simulink model "CSvRTHS_Client"  (R2020b)
settings: Solver=ode8  StartTime=0.0  StopTime=inf  FixedStep=samplePeriod  RelTol=1e-3  AbsTol=1e-6  EnableMultiTasking=on
PreLoadFcn:
  | initializeSimulation;
InitFcn:
  | clear('all');
  | initializeSimulation;
values from neighbouring files (symbols this model uses):
  adaptivegain = diag(10.^[6.03 4.23 1.48 -1.10])    [initializeSimulation.m]
  Area = 0.751    [initializeSimulation.m]
  Be = 95958    [initializeSimulation.m]
  Cl = 5.89e-6    (= 5.89e-06)    [initializeSimulation.m]
  coef = 1.0    (= 1)    [initializeSimulation.m]
  damperB = 0    [initializeSimulation.m]
  damperCanon = 1    [initializeSimulation.m]
  Derivadas = [u;dudt;dudt2;dudt3]    [initializeSimulation.m]
  forceCanon = 1    [initializeSimulation.m]
  frictionB = 0    [initializeSimulation.m]
  Gsnsr_DT = 1    [initializeSimulation.m]
  Gsnsr_FT = 1    [initializeSimulation.m]
  Kc = 1.36e-5    (= 1.36e-05)    [initializeSimulation.m]
  Kp = 3.0    (= 3)    [initializeSimulation.m]
  Kq = 23.01    [initializeSimulation.m]
  kv = 1    [initializeSimulation.m]
  lengthCanon = 1    [initializeSimulation.m]
  max_amb = [amb0max,amb1max,amb2max,amb3max]*1e15    [initializeSimulation.m]
  maxDisplB = (stroke2B + endLength2B) * lengthCanon    (= 42)    [initializeSimulation.m]
  maxVelocB = (maxFlowB * flowCanon / (area1B * areaCanon)) / velocCanon    [initializeSimulation.m]
  me = 0.023/1000    (= 2.3e-05)    [initializeSimulation.m]
  min_amb = [amb0min,amb1min,amb2min,amb3min]    [initializeSimulation.m]
  minDisplB = -(stroke1B + endLength1B) * lengthCanon    (= -42)    [initializeSimulation.m]
  minVelocB = -(maxFlowB * flowCanon / (area2B * areaCanon)) / velocCanon    [initializeSimulation.m]
  samplePeriod = 0.5/1024    (= 0.00048828125)    [initializeSimulation.m]
  sat_limit_lower = -3.8    [initializeSimulation.m]
  sat_limit_upper = +3.8    (= 3.8)    [initializeSimulation.m]
  Seed_snr = rng(seed)    [initializeSimulation.m]
  staticForceB = 0    [initializeSimulation.m]
  tauv = 0.00332    [initializeSimulation.m]
  velocCanon = 1    [initializeSimulation.m]
  Vt = 48.66    [initializeSimulation.m]
  yieldDisplB = 0.1    [initializeSimulation.m]
undefined symbols (not defined in the file or in its folder): denfilter, DiscIntNeverNeededParam, HybridCtrlParameters, numfilter
libraries: simulink x7, dsparch4 x1, sldrtlib x1
settings Model: ExtModeTrigMode=oneshot  ExtModeArmWhenConnect=off  ExtModeAutoUpdateStatusClock=off  Creator=Andreas Schellenberg  LastModifiedBy=diego.mera
settings SolverCC: AutoScaleAbsTol=off
settings DataIOCC: LimitDataPoints=on  SaveFormat=Array  SaveOutput=off  ReturnWorkspaceOutputs=off  SignalLoggingName=sigsOut
settings OptimizationCC: ExpressionDepthLimit=2147483647  InitFltsAndDblsToZero=on  LifeSpan=inf
settings DebuggingCC: SaveWithParameterizedLinksMsg=none  CheckSSInitialOutputMsg=off  UnderspecifiedInitializationDetection=Classic  MergeDetectMultiDrivingBlocksExec=none  MultiTaskDSMMsg=warning  MultiTaskCondExecSysMsg=none  StateNameClashWarn=warning  SFUnexpectedBacktrackingDiag=warning  SFNoUnconditionalDefaultTransitionDiag=warning  SFExecutionAtInitializationDiag=none  ArithmeticOperatorsInVariantConditions=warning
settings HardwareCC: ProdBitPerPointer=32  ProdBitPerSizeT=32  ProdBitPerPtrDiffT=32  ProdLargestAtomicFloat=None  ProdIntDivRoundTo=Undefined  ProdEndianess=Unspecified  ProdWordSize=32  ProdHWDeviceType=32-bit Generic  TargetUnknown=on
settings ModelReferenceCC: PropagateSignalLabelsOutOfModel=off
settings SFSimCC: SimCustomHeaderCode="#include \"PredictorCorrector.h\""  SimUserSources=PredictorCorrector.c  SimUseLocalCustomCode=off  SimParseCustomCode=off  CustomCodeUndefinedFunction=UseInterfaceOnly
settings RTWCC: RTWUseLocalCustomCode=off
settings CodeAppCC: StateflowObjectComments=on
settings GRTTargetCC: TargetFcnLib=ansi_tfl_tmw.mat  TargetLangStandard=C89/C90 (ANSI)  CombineOutputUpdateFcns=off  GRTInterface=on
settings ConfigComp: CovMetricSettings=dw  CovSaveCumulativeToWorkspaceVar=on  CovSaveSingleToWorkspaceVar=on  CovExternalEMLEnable=off  CovSFcnEnable=off

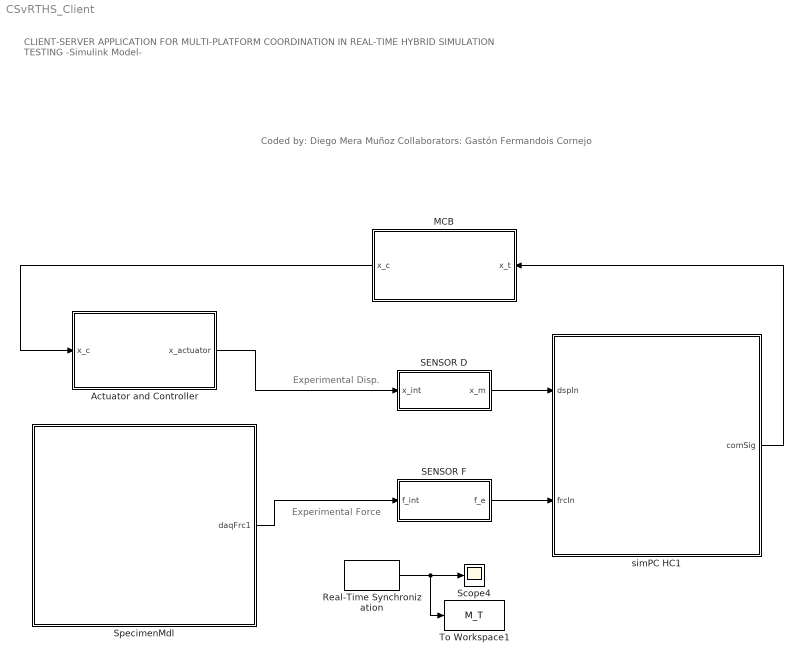
== system CSvRTHS_Client ==
  note: CLIENT-SERVER APPLICATION FOR MULTI-PLATFORM COORDINATION IN REAL-TIME HYBRID SIMULATION TESTING
      | -Simulink Model-
  note: Coded by: Diego Mera Muñoz
      | Collaborators: Gastón Fermandois Cornejo
  note: Experimental Force
  note: Experimental Disp.
  Actuator and Controller : Subsystem
      mask Display: disp('ACTUATOR\nMODEL')
  MCB : Subsystem
      mask Display: disp('ADAPTIVE\nMODEL-BASED\nCOMPENSATION')
  Real-Time Synchronization : sldrtlib/Real-Time Synchronization  SampleTime=0.5/1024  MaxMissedTicks=1000000  ShowMissedTicks=on  YieldWhenWaiting=off
  SENSOR D : Subsystem
  SENSOR F : Subsystem
  Scope4 : Scope
  SpecimenMdl : Subsystem
      mask Display: disp('EXPERIMENTAL\nSUBSTRUCTURE')
  To Workspace1 : ToWorkspace  VariableName=M_T  SaveFormat=Timeseries  SampleTime=-1
  simPC HC1 : Subsystem  mask(Hybrid Controller: D2/D2){nDOF=HybridCtrlParameters.nDOF, upFact=HybridCtrlParameters.upFact, dtInt=HybridCtrlParameters.dtInt, dtSim=HybridCtrlParameters.dtSim, dtCon=HybridCtrlParameters.dtCon, N=HybridCtrlParameters.N, iDelay=HybridCtrlParameters.iDelay}
      mask prompts: nDOF "Number of DOF: nDOF"; upFact "Upsample Factor: upFact"; dtInt "Integration time step: dtInt"; dtSim "Simulation time step: dtSim"; dtCon "Controller time step: dtCon"; N "Number of substeps: N"; iDelay "Number of delay steps: iDelay"
      mask help: Hybrid Controller using C0-continuous quadratic Lagrange interpolation for prediction and correction
      mask Display: disp('NUMERICAL\nSUBSTRUCTURE')
  wires:
  SENSOR F/1("f_e ") -> simPC HC1/2(frcIn)
  MCB/1(x_c) -> Actuator and Controller/1(x_c)
  SpecimenMdl/1(daqFrc1) -> SENSOR F/1(f_int)
  SENSOR D/1(x_m) -> simPC HC1/1(dspIn)
  simPC HC1/1(comSig) -> MCB/1(x_t)
  Actuator and Controller/1(x_actuator) -> SENSOR D/1(x_int)
  Real-Time Synchronization/1 -> To Workspace1/1, Scope4/1

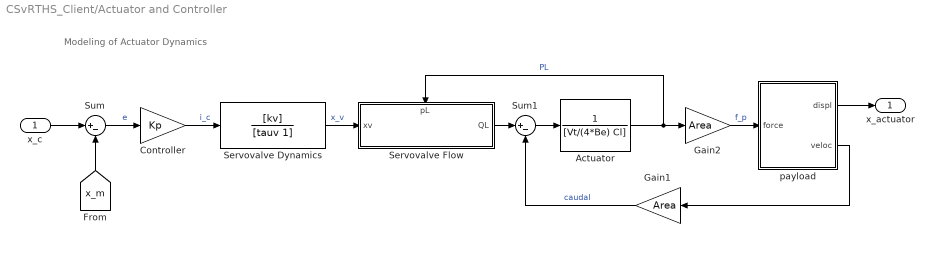
== system CSvRTHS_Client/Actuator and Controller ==
  note: Modeling of Actuator Dynamics
  x_c : Inport
  Actuator : TransferFcn  Denominator=[Vt/(4*Be) Cl]
      mask Display: image(imread('actuator.PNG'));
  Controller : Gain  Gain=Kp
  Gain1 : Gain  Gain=Area
  Gain2 : Gain  Gain=Area
  Servovalve Dynamics : TransferFcn  Numerator=[kv]  Denominator=[tauv 1]
      mask Display: image(imread('servo2.PNG'));
  Servovalve Flow : Subsystem
      settings: PortSchema="{\"entries\":[{\"content\":{\"sides\":[{\"content\":{\"connectorIds\":[\"In1\"]},\"type\":\"ConnectorPlacement.EquallySpacedRectSide\",\"uuid\":\"f3a8b7d5-d784-462c-bc82-60644eee5a75\"},{\"content\":{\"connectorIds\":[\"Out1\"],\"side\":\"RIGHT\"},\"type\":\"ConnectorPlacement.EquallySpacedRectSide\",\"uuid\":\"5e6f1f83-a632-4bc9-a761-43cae998e77f\"},{\"content\":{\"connectorIds\":[\"In2\"],\"side\":\"TOP\"},\"type\":\"ConnectorPlacement.EquallySpacedRectSide\",\"uuid\":\"989b0903-e260-4847-946f-0ac5d5e511f7\"}]},\"type\":\"ConnectorPlacement.EquallySpacedConnector\",\"uuid\":\"5619e211-faa3-4076-b1a0-b20862ba0eaa\"}],\"packageUris\":[\"http://schema.mathworks.com/mf0/Connector/19700101\"],\"version\":\"1.0\"}"
      mask Display: image(imread('servo.PNG'));
  Sum : Sum  Inputs=|+-
  Sum1 : Sum  Inputs=|+-
  payload : Subsystem
  x_actuator : Outport  VectorParamsAs1DForOutWhenUnconnected=off
  wires:
  Sum1/1 -> Actuator/1
  Sum/1 -> Controller/1  "e"
  Servovalve Dynamics/1 -> Servovalve Flow/1(xv)  "x_v"
  Servovalve Flow/1(QL) -> Sum1/1
  Gain1/1 -> Sum1/2  "caudal"
  Actuator/1 -> Gain2/1, Servovalve Flow/2(pL)  "PL"
  payload/1(displ) -> x_actuator/1
  Controller/1 -> Servovalve Dynamics/1  "i_c"
  payload/2(veloc) -> Gain1/1
  Gain2/1 -> payload/1(force)  "f_p"
  x_c/1 -> Sum/1
  [x_m] -> Sum/2

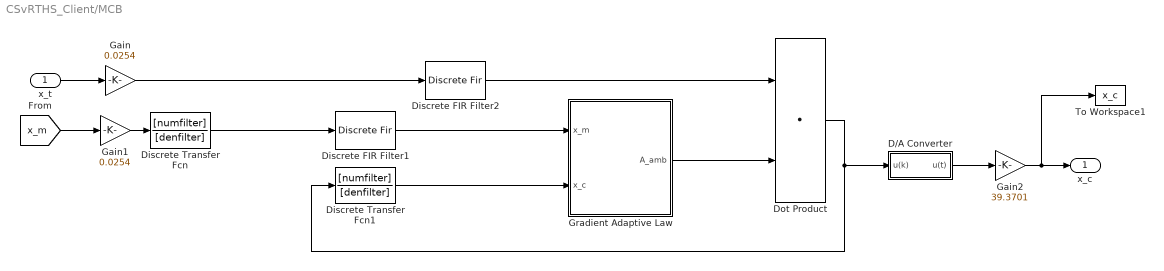
== system CSvRTHS_Client/MCB ==
  x_t : Inport
  D/A Converter : Subsystem
  Discrete Transfer Fcn : DiscreteTransferFcn  Numerator=[numfilter]  Denominator=[denfilter]
  Discrete Transfer Fcn1 : DiscreteTransferFcn  Numerator=[numfilter]  Denominator=[denfilter]
  Discrete FIR Filter1 : DiscreteFir  Coefficients=Derivadas
  Discrete FIR Filter2 : DiscreteFir  Coefficients=Derivadas
  Dot Product : DotProduct  InputSameDT=on  OutDataTypeStr=Inherit: Inherit via internal rule
  Gain : Gain  Gain=0.0254
  Gain1 : Gain  Gain=0.0254
  Gain2 : Gain  Gain=39.3701
  Gradient Adaptive Law : Subsystem
  To Workspace1 : ToWorkspace  VariableName=x_c  SaveFormat=Timeseries  SampleTime=-1
  x_c : Outport  VectorParamsAs1DForOutWhenUnconnected=off
  wires:
  Gradient Adaptive Law/1(A_amb) -> Dot Product/2
  Discrete FIR Filter1/1 -> Gradient Adaptive Law/1(x_m)
  Discrete Transfer Fcn1/1 -> Gradient Adaptive Law/2(x_c)
  [x_m] -> Gain1/1
  Discrete Transfer Fcn/1 -> Discrete FIR Filter1/1
  x_t/1 -> Gain/1
  Dot Product/1 -> D/A Converter/1(u(k)), Discrete Transfer Fcn1/1
  Discrete FIR Filter2/1 -> Dot Product/1
  D/A Converter/1(u(t)) -> Gain2/1
  Gain1/1 -> Discrete Transfer Fcn/1
  Gain/1 -> Discrete FIR Filter2/1
  Gain2/1 -> To Workspace1/1, x_c/1

== system CSvRTHS_Client/SENSOR D ==
  x_int : Inport
  Sensor Noise : simulink/Sources/Band-Limited White Noise  Cov=rms_noise_DT  Ts=samplePeriod  seed=double(Seed_snr.Seed)
  Sensor Gain LVDT : Gain  Gain=Gsnsr_DT  SaturateOnIntegerOverflow=on  OutDataTypeStr=Inherit: Same as input  ParamDataTypeStr=Inherit: Same as input
  Sum : Sum  Inputs=|++  InputSameDT=on  SaturateOnIntegerOverflow=on  OutDataTypeStr=Inherit: Same as first input
  To Workspace : ToWorkspace  VariableName=x_m  SaveFormat=Timeseries  SampleTime=-1
  x_m : Outport
  tag scope: x_m=global
  wires:
  Sensor Gain LVDT/1 -> Sum/1
  Sensor Noise/1 -> Sum/2
  x_int/1 -> Sensor Gain LVDT/1
  Sum/1 -> [x_m], x_m/1, To Workspace/1

== system CSvRTHS_Client/SENSOR F ==
  f_int : Inport
  Sensor Noise1 : simulink/Sources/Band-Limited White Noise  Cov=rms_noise_FT  Ts=samplePeriod  seed=double(Seed_snr.Seed)
  Sensor Gain LOAD CELL : Gain  Gain=Gsnsr_FT  SaturateOnIntegerOverflow=on  OutDataTypeStr=Inherit: Same as input  ParamDataTypeStr=Inherit: Same as input
  Sum1 : Sum  Inputs=|++  InputSameDT=on  SaturateOnIntegerOverflow=on  OutDataTypeStr=Inherit: Same as first input
  To Workspace1 : ToWorkspace  VariableName=f_m  SaveFormat=Timeseries  SampleTime=-1
  "f_e " : Outport
  wires:
  Sensor Gain LOAD CELL/1 -> Sum1/1
  Sum1/1 -> To Workspace1/1, "f_e "/1
  Sensor Noise1/1 -> Sum1/2
  f_int/1 -> Sensor Gain LOAD CELL/1

== system CSvRTHS_Client/SpecimenMdl ==
  note: Experimental Force
  note: Experimental Disp
  S-Function : S-Function  FunctionName=SFun_GenericClient  Parameters=ipAddr,ipPort,dataSize  SFunctionDeploymentMode=off  EnableBusSupport=off  mask(GenericClient Element){ipAddr=127.0.0.1, ipPort=8093, dataSize=256}
      mask prompts: ipAddr "IP Address of Server"; ipPort "IP Port Number of Server"; dataSize "Size of Data Arrays"
      mask Display: disp('GenericClient\nElement');
  Scope1 : Scope
  Terminator1 : Terminator
  daqFrc1 : Outport
  tag scope: ch3b=global
  wires:
  [ch3a] -> S-Function/1
  S-Function/1 -> Terminator1/1
  S-Function/2 -> daqFrc1/1, [ch3b], Scope1/1

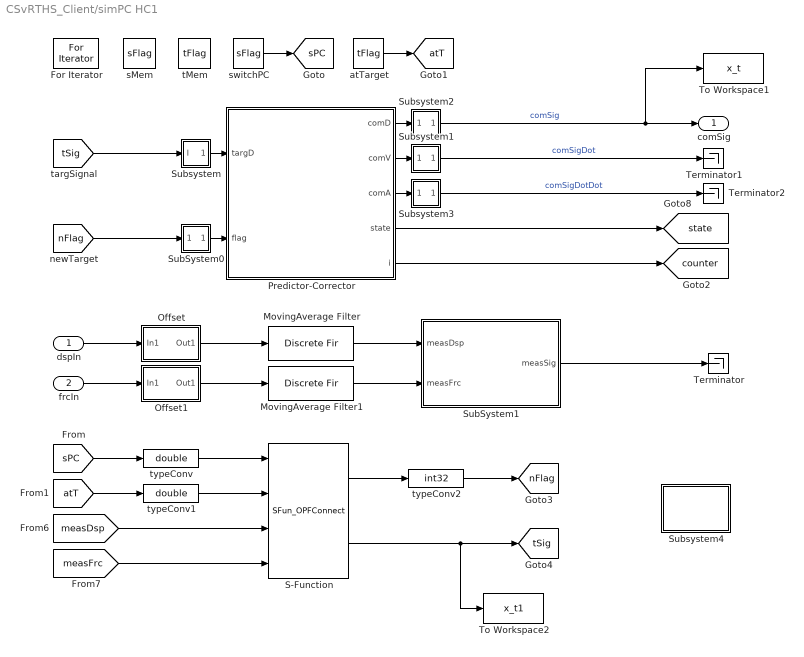
== system CSvRTHS_Client/simPC HC1 ==
  dspIn : Inport
  frcIn : Inport  Port=2
  For Iterator : ForIterator  IterationLimit=upFact  ShowIterationPort=off
  MovingAverage Filter : DiscreteFir  Coefficients=1/numSample*ones(1,numSample)  mask(Moving Average Filter){numSample=1}
      mask prompts: numSample "Number of Samples: numSample"
      mask help:
      | Moving average filter by using discrete FIR filter.
      | Set numSample = 1 for no filtering.
      mask Display: fprintf('MovingAverage\nFilter')
  MovingAverage Filter1 : DiscreteFir  Coefficients=1/numSample*ones(1,numSample)  mask(Moving Average Filter){numSample=1}
      mask prompts: numSample "Number of Samples: numSample"
      mask help:
      | Moving average filter by using discrete FIR filter.
      | Set numSample = 1 for no filtering.
      mask Display: fprintf('MovingAverage\nFilter')
  Offset : Subsystem  mask(Signal Offset){nS=nDOF, nOffset=-1}
      mask prompts: nS "Number of Signals: nS"; nOffset "Number of samples to initialize offset: nOffset"
      mask help:
      | Offset signal by average of signal over initial number of samples.
      | Set nOffset = -1 for no signal offset.
      mask Display: fprintf('Signal\nOffset')
  Offset1 : Subsystem  mask(Signal Offset){nS=nDOF, nOffset=-1}
      mask prompts: nS "Number of Signals: nS"; nOffset "Number of samples to initialize offset: nOffset"
      mask help:
      | Offset signal by average of signal over initial number of samples.
      | Set nOffset = -1 for no signal offset.
      mask Display: fprintf('Signal\nOffset')
  Predictor-Corrector : Stateflow chart  TreatAsAtomicUnit=on
  S-Function : S-Function  FunctionName=SFun_OPFConnect  Parameters=ipPort  SFunctionDeploymentMode=off  EnableBusSupport=off  mask(OpenFresco Connect){ipPort=8090}
      mask prompts: ipPort "IP Port Number of Server"
      mask Display: disp('OpenFresco\nConnect');
  SubSystem0 : Subsystem
      mask Display: disp('I/O')
  SubSystem1 : Subsystem
  Subsystem : Subsystem
      mask Display: disp('I/O')
  Subsystem1 : Subsystem
      mask Display: disp('I/O')
  Subsystem2 : Subsystem
      mask Display: disp('I/O')
  Subsystem3 : Subsystem
      mask Display: disp('I/O')
  Subsystem4 : Subsystem
      mask Display: disp('Scopes')
  Terminator : Terminator
  Terminator1 : Terminator
  Terminator2 : Terminator
  To Workspace1 : ToWorkspace  VariableName=x_t  SaveFormat=Timeseries  SampleTime=-1
  To Workspace2 : ToWorkspace  VariableName=x_t1  SaveFormat=Timeseries  SampleTime=-1
  atTarget : DataStoreRead  DataStoreName=tFlag
  sMem : DataStoreMemory  DataStoreName=sFlag  ShowAdditionalParam=off  OutDataTypeStr=int32
  switchPC : DataStoreRead  DataStoreName=sFlag
  tMem : DataStoreMemory  DataStoreName=tFlag  ShowAdditionalParam=off  OutDataTypeStr=int32
  typeConv : DataTypeConversion  OutDataTypeStr=double  RndMeth=Round  SaturateOnIntegerOverflow=on
  typeConv1 : DataTypeConversion  OutDataTypeStr=double  RndMeth=Round  SaturateOnIntegerOverflow=on
  typeConv2 : DataTypeConversion  OutDataTypeStr=int32  RndMeth=Round  SaturateOnIntegerOverflow=on
  comSig : Outport
  tag scope: atT=global, counter=global, nFlag=global, sPC=global, state=global, tSig=global
  wires:
  SubSystem0/1(Out) -> Predictor-Corrector/2(flag)
  [nFlag] -> SubSystem0/1(In)
  [tSig] -> Subsystem/1(I)
  [sPC] -> typeConv/1
  [atT] -> typeConv1/1
  S-Function/1 -> typeConv2/1
  S-Function/2 -> [tSig], To Workspace2/1
  Subsystem/1(O) -> Predictor-Corrector/1(targD)
  Subsystem2/1(Out) -> comSig/1, To Workspace1/1  "comSig"
  switchPC/1 -> [sPC]
  atTarget/1 -> [atT]
  Predictor-Corrector/1(comD) -> Subsystem2/1(In)
  Subsystem1/1(Out) -> Terminator1/1  "comSigDot"
  Predictor-Corrector/2(comV) -> Subsystem1/1(In)
  Subsystem3/1(Out) -> Terminator2/1  "comSigDotDot"
  Predictor-Corrector/3(comA) -> Subsystem3/1(In)
  frcIn/1 -> Offset1/1(In1)
  SubSystem1/1(measSig) -> Terminator/1
  dspIn/1 -> Offset/1(In1)
  MovingAverage Filter/1 -> SubSystem1/1(measDsp)
  MovingAverage Filter1/1 -> SubSystem1/2(measFrc)
  Offset/1(Out1) -> MovingAverage Filter/1
  Offset1/1(Out1) -> MovingAverage Filter1/1
  Predictor-Corrector/5(i) -> [counter]
  Predictor-Corrector/4(state) -> [state]
  [measFrc] -> S-Function/4
  [measDsp] -> S-Function/3
  typeConv/1 -> S-Function/1
  typeConv1/1 -> S-Function/2
  typeConv2/1 -> [nFlag]

== system CSvRTHS_Client/Actuator and Controller/Servovalve Flow ==
  xv : Inport
  pL : Inport  Port=2
  Gain : Gain  Gain=Kq
  Gain1 : Gain  Gain=Kc
  Subtract : Sum  Inputs=+-
  QL : Outport
  wires:
  Gain1/1 -> Subtract/2
  pL/1 -> Gain1/1
  Subtract/1 -> QL/1
  Gain/1 -> Subtract/1
  xv/1 -> Gain/1

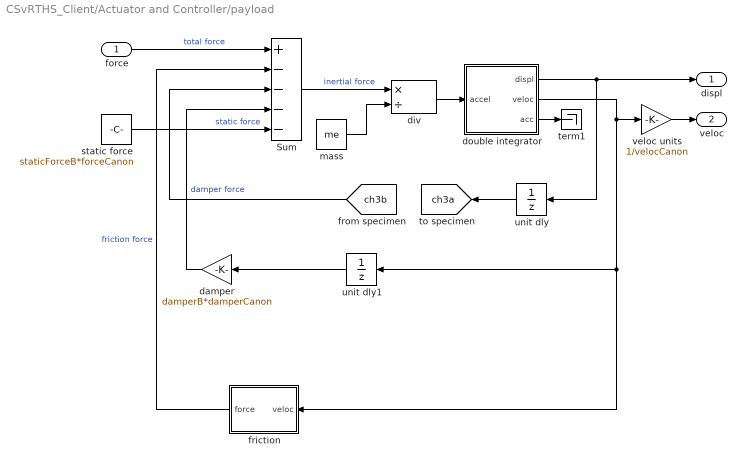
== system CSvRTHS_Client/Actuator and Controller/payload ==
  force : Inport
  Sum : Sum  Inputs=+----  InputSameDT=on  SaturateOnIntegerOverflow=on  OutDataTypeStr=Inherit: Same as first input
  damper : Gain  Gain=damperB*damperCanon  SaturateOnIntegerOverflow=on  OutDataTypeStr=Inherit: Same as input  ParamDataTypeStr=Inherit: Same as input
  div : Product  Inputs=*/  InputSameDT=on  SaturateOnIntegerOverflow=on  OutDataTypeStr=Inherit: Same as first input
  double integrator : Subsystem
  friction : Subsystem  mask{friction=frictionB*forceCanon, yieldDispl=yieldDisplB*lengthCanon, hysteresis=0}
      mask prompts: friction "Sliding friction"; yieldDispl "Equiv. yield displacement (in)"; hysteresis "Hysteresis constant"
  mass : Constant  Value=me
  static force : Constant  Value=staticForceB*forceCanon
  term1 : Terminator
  unit dly : UnitDelay  SampleTime=-1  HasFrameUpgradeWarning=on
  unit dly1 : UnitDelay  SampleTime=-1  HasFrameUpgradeWarning=on
  veloc units : Gain  Gain=1/velocCanon  SaturateOnIntegerOverflow=on  OutDataTypeStr=Inherit: Same as input  ParamDataTypeStr=Inherit: Same as input
  displ : Outport
  veloc : Outport  Port=2
  tag scope: ch3a=global
  wires:
  unit dly1/1 -> damper/1
  unit dly/1 -> [ch3a]
  damper/1 -> Sum/4  "damper force"
  static force/1 -> Sum/5  "static force"
  double integrator/2(veloc) -> unit dly1/1, friction/1(veloc), veloc units/1
  double integrator/1(displ) -> unit dly/1, displ/1
  div/1 -> double integrator/1(accel)
  double integrator/3(acc) -> term1/1
  mass/1 -> div/2
  force/1 -> Sum/1  "total force"
  Sum/1 -> div/1  "inertial force"
  veloc units/1 -> veloc/1
  friction/1(force) -> Sum/2  "friction force"
  [ch3b] -> Sum/3

== system CSvRTHS_Client/MCB/D//A Converter ==
  u(k) : Inport
  Quantizer : Quantizer  QuantizationInterval=quantize_int
  Saturation : Saturate  UpperLimit=sat_limit_upper  LowerLimit=sat_limit_lower
  u(t) : Outport  VectorParamsAs1DForOutWhenUnconnected=off
  wires:
  Saturation/1 -> u(t)/1
  Quantizer/1 -> Saturation/1
  u(k)/1 -> Quantizer/1

== system CSvRTHS_Client/MCB/Gradient Adaptive Law ==
  x_m : Inport
  x_c : Inport  Port=2
  Constant4 : Constant  Value=adaptivegain
  Integrator : Integrator  InitialCondition=A_amb_i'
  Saturation : Saturate  UpperLimit=[max_amb]  LowerLimit=min_amb
  To Workspace : ToWorkspace  VariableName=amb  SaveFormat=Timeseries  SampleTime=-1
  gradiente_adaptive_law : MATLAB Function  TreatAsAtomicUnit=on
  A_amb : Outport  VectorParamsAs1DForOutWhenUnconnected=off
  wires:
  Saturation/1 -> gradiente_adaptive_law/3(amb_a), To Workspace/1, A_amb/1
  Integrator/1 -> Saturation/1
  x_c/1 -> gradiente_adaptive_law/2(x_c)
  Constant4/1 -> gradiente_adaptive_law/4(adaptivegain)
  gradiente_adaptive_law/1(A_ambp) -> Integrator/1
  x_m/1 -> gradiente_adaptive_law/1(x_m)

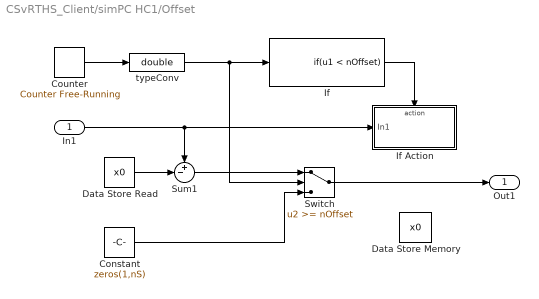
== system CSvRTHS_Client/simPC HC1/Offset ==
  In1 : Inport
  Constant : Constant  Value=zeros(1,nS)
  Counter : simulink/Sources/Counter Free-Running  NumBits=32  tsamp=-1
  Data Store Memory : DataStoreMemory  DataStoreName=x0  InitialValue=zeros(1,nS)  ShowAdditionalParam=off  OutDataTypeStr=double
  Data Store Read : DataStoreRead  DataStoreName=x0
  If : If  IfExpression=u1 < nOffset  ShowElse=off
  If Action : Subsystem  TreatAsAtomicUnit=on
  Sum1 : Sum  Inputs=+-|  InputSameDT=on  SaturateOnIntegerOverflow=on  OutDataTypeStr=Inherit: Same as first input
  Switch : Switch  Threshold=nOffset  SaturateOnIntegerOverflow=on  InputSameDT=on
  typeConv : DataTypeConversion  OutDataTypeStr=double  RndMeth=Round  SaturateOnIntegerOverflow=on
  Out1 : Outport
  wires:
  Switch/1 -> Out1/1
  Sum1/1 -> Switch/1
  Data Store Read/1 -> Sum1/2
  In1/1 -> If Action/1(In1), Sum1/1
  Constant/1 -> Switch/3
  Counter/1 -> typeConv/1
  If/1 -> If Action/Action
  typeConv/1 -> Switch/2, If/1

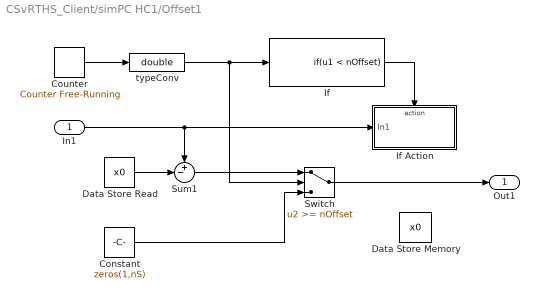
== system CSvRTHS_Client/simPC HC1/Offset1 ==
  In1 : Inport
  Constant : Constant  Value=zeros(1,nS)
  Counter : simulink/Sources/Counter Free-Running  NumBits=32  tsamp=-1
  Data Store Memory : DataStoreMemory  DataStoreName=x0  InitialValue=zeros(1,nS)  ShowAdditionalParam=off  OutDataTypeStr=double
  Data Store Read : DataStoreRead  DataStoreName=x0
  If : If  IfExpression=u1 < nOffset  ShowElse=off
  If Action : Subsystem  TreatAsAtomicUnit=on
  Sum1 : Sum  Inputs=+-|  InputSameDT=on  SaturateOnIntegerOverflow=on  OutDataTypeStr=Inherit: Same as first input
  Switch : Switch  Threshold=nOffset  SaturateOnIntegerOverflow=on  InputSameDT=on
  typeConv : DataTypeConversion  OutDataTypeStr=double  RndMeth=Round  SaturateOnIntegerOverflow=on
  Out1 : Outport
  wires:
  Switch/1 -> Out1/1
  Sum1/1 -> Switch/1
  Data Store Read/1 -> Sum1/2
  In1/1 -> If Action/1(In1), Sum1/1
  Constant/1 -> Switch/3
  Counter/1 -> typeConv/1
  If/1 -> If Action/Action
  typeConv/1 -> Switch/2, If/1

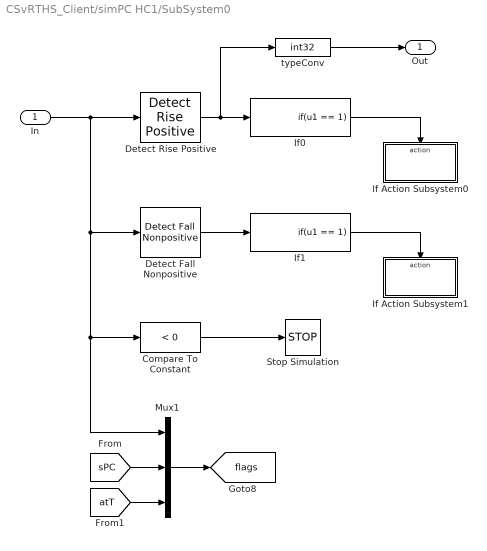
== system CSvRTHS_Client/simPC HC1/SubSystem0 ==
  In : Inport
  Compare To Constant : simulink/Logic and Bit Operations/Compare To Constant  relop=<  const=0  OutDataTypeStr=boolean
  Detect Fall Nonpositive : simulink/Logic and Bit Operations/Detect Fall Nonpositive  vinit=0  OutDataTypeStr=uint8
      settings: SourceProductBaseCode=SL
  Detect Rise Positive : simulink/Logic and Bit Operations/Detect Rise Positive  vinit=0  OutDataTypeStr=uint8
  If Action Subsystem0 : Subsystem  TreatAsAtomicUnit=on
  If Action Subsystem1 : Subsystem  TreatAsAtomicUnit=on
  If0 : If  IfExpression=u1 == 1  ShowElse=off
  If1 : If  IfExpression=u1 == 1  ShowElse=off
  Mux1 : Mux  Inputs=3
  Stop Simulation : Stop
  typeConv : DataTypeConversion  OutDataTypeStr=int32  RndMeth=Round  SaturateOnIntegerOverflow=on
  Out : Outport
  tag scope: flags=global
  wires:
  Detect Rise Positive/1 -> If0/1, typeConv/1
  Detect Fall Nonpositive/1 -> If1/1
  If1/1 -> If Action Subsystem1/Action
  If0/1 -> If Action Subsystem0/Action
  typeConv/1 -> Out/1
  Mux1/1 -> [flags]
  [sPC] -> Mux1/2
  [atT] -> Mux1/3
  In/1 -> Detect Rise Positive/1, Detect Fall Nonpositive/1, Compare To Constant/1, Mux1/1
  Compare To Constant/1 -> Stop Simulation/1

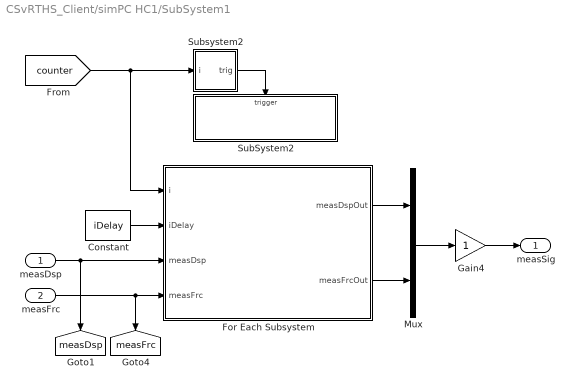
== system CSvRTHS_Client/simPC HC1/SubSystem1 ==
  measDsp : Inport
  measFrc : Inport  Port=2
  Constant : Constant  Value=iDelay
  For Each Subsystem : Subsystem  TreatAsAtomicUnit=on
  Gain4 : Gain  SaturateOnIntegerOverflow=on  OutDataTypeStr=Inherit: Same as input  ParamDataTypeStr=Inherit: Same as input
  Mux : Mux  Inputs=2
  SubSystem2 : Subsystem  TreatAsAtomicUnit=on
  Subsystem2 : Subsystem
  measSig : Outport
  tag scope: measDsp=global, measFrc=global
  wires:
  Subsystem2/1(trig) -> SubSystem2/Trigger
  [counter] -> Subsystem2/1(i), For Each Subsystem/1(i)
  Gain4/1 -> measSig/1
  Constant/1 -> For Each Subsystem/2(iDelay)
  measDsp/1 -> [measDsp], For Each Subsystem/3(measDsp)
  measFrc/1 -> For Each Subsystem/4(measFrc), [measFrc]
  For Each Subsystem/1(measDspOut) -> Mux/1
  For Each Subsystem/2(measFrcOut) -> Mux/2
  Mux/1 -> Gain4/1

== system CSvRTHS_Client/simPC HC1/Subsystem ==
  I : Inport  PortDimensions=nDOF
  Dummy Aug : Mux  Inputs=[nDOF 1]
  Dummy Zero : Constant  Value=0  OutDataTypeStr=double  SampleTime=-1
  O : Outport  PortDimensions=nDOF+1
  tag scope: targSig=global
  wires:
  Dummy Zero/1 -> Dummy Aug/2
  I/1 -> Dummy Aug/1, [targSig]
  Dummy Aug/1 -> O/1

== system CSvRTHS_Client/simPC HC1/Subsystem1 ==
  In : Inport  PortDimensions=nDOF+1
  Dummy Trn : Demux  Outputs=[nDOF 1]
  Terminator3 : Terminator
  Out : Outport  PortDimensions=nDOF
  wires:
  Dummy Trn/2 -> Terminator3/1
  Dummy Trn/1 -> Out/1
  In/1 -> Dummy Trn/1

== system CSvRTHS_Client/simPC HC1/Subsystem2 ==
  In : Inport  PortDimensions=nDOF+1
  Dummy Trn : Demux  Outputs=[nDOF 1]
  Terminator3 : Terminator
  Out : Outport  PortDimensions=nDOF
  tag scope: comSig=global
  wires:
  Dummy Trn/2 -> Terminator3/1
  Dummy Trn/1 -> Out/1, [comSig]
  In/1 -> Dummy Trn/1

== system CSvRTHS_Client/simPC HC1/Subsystem3 ==
  In : Inport  PortDimensions=nDOF+1
  Dummy Trn : Demux  Outputs=[nDOF 1]
  Terminator3 : Terminator
  Out : Outport  PortDimensions=nDOF
  wires:
  Dummy Trn/2 -> Terminator3/1
  Dummy Trn/1 -> Out/1
  In/1 -> Dummy Trn/1

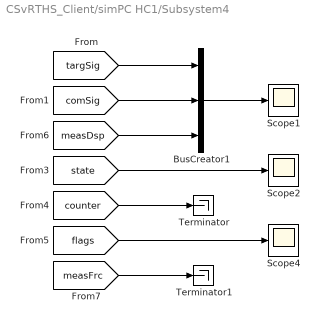
== system CSvRTHS_Client/simPC HC1/Subsystem4 ==
  BusCreator1 : BusCreator  Inputs=3
  Scope1 : Scope
  Scope2 : Scope
  Scope4 : Scope
  Terminator : Terminator
  Terminator1 : Terminator
  wires:
  [targSig] -> BusCreator1/1
  [comSig] -> BusCreator1/2
  [flags] -> Scope4/1
  [measDsp] -> BusCreator1/3
  BusCreator1/1 -> Scope1/1
  [state] -> Scope2/1
  [counter] -> Terminator/1
  [measFrc] -> Terminator1/1

== system CSvRTHS_Client/Actuator and Controller/payload/double integrator ==
  accel : Inport
  Analog Filter Design : dsparch4/Analog Filter Design  method=Butterworth  filttype=Lowpass  N=1  Wlo=30  Whi=80  Rp=2  Rs=40
  displ gen : DiscreteIntegrator  IntegratorMethod=Integration: Backward Euler  SampleTime=0.5/1024  LimitOutput=on  UpperSaturationLimit=maxDisplB*coef  LowerSaturationLimit=minDisplB*coef  ShowSaturationPort=on  ICPrevOutput=DiscIntNeverNeededParam  ICPrevScaledInput=DiscIntNeverNeededParam
  veloc gen : Subsystem  mask{maxVeloc=maxVelocB*velocCanon*coef, minVeloc=minVelocB*velocCanon*coef, maxDispl=maxDisplB*coef, minDispl=minDisplB*coef}
      mask prompts: maxVeloc "Max velocity"; minVeloc "Min velocity"; maxDispl "Max displacement"; minDispl "Min displacement"
  displ : Outport
  veloc : Outport  Port=2
  acc : Outport  Port=3
  wires:
  accel/1 -> acc/1, veloc gen/1(accel)
  veloc gen/1(veloc) -> veloc/1, displ gen/1
  displ gen/1 -> Analog Filter Design/1, veloc gen/2(displ)
  displ gen/2 -> veloc gen/3(reset)
  Analog Filter Design/1 -> displ/1

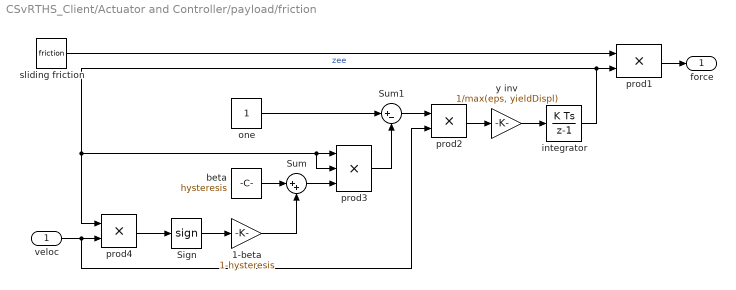
== system CSvRTHS_Client/Actuator and Controller/payload/friction ==
  veloc : Inport
  1-beta : Gain  Gain=1-hysteresis  SaturateOnIntegerOverflow=on  OutDataTypeStr=Inherit: Same as input  ParamDataTypeStr=Inherit: Same as input
  Sign : Signum
  Sum : Sum  Inputs=|++  SaturateOnIntegerOverflow=on
  Sum1 : Sum  Inputs=|+-  SaturateOnIntegerOverflow=on
  beta : Constant  Value=hysteresis
  integrator : DiscreteIntegrator  SampleTime=-1  LimitOutput=on  UpperSaturationLimit=1  LowerSaturationLimit=-1  ICPrevOutput=DiscIntNeverNeededParam  ICPrevScaledInput=DiscIntNeverNeededParam
  one : Constant
  prod1 : Product  InputSameDT=on  SaturateOnIntegerOverflow=on  OutDataTypeStr=Inherit: Same as first input
  prod2 : Product  InputSameDT=on  SaturateOnIntegerOverflow=on  OutDataTypeStr=Inherit: Same as first input
  prod3 : Product  Inputs=3  InputSameDT=on  SaturateOnIntegerOverflow=on  OutDataTypeStr=Inherit: Same as first input
  prod4 : Product  InputSameDT=on  SaturateOnIntegerOverflow=on  OutDataTypeStr=Inherit: Same as first input
  sliding friction : Constant  Value=friction
  y inv : Gain  Gain=1/max(eps, yieldDispl)  SaturateOnIntegerOverflow=on  OutDataTypeStr=Inherit: Same as input  ParamDataTypeStr=Inherit: Same as input
  force : Outport
  wires:
  integrator/1 -> prod3/2, prod3/1, prod4/1, prod1/2  "zee"
  y inv/1 -> integrator/1
  prod2/1 -> y inv/1
  Sum1/1 -> prod2/1
  prod3/1 -> Sum1/2
  one/1 -> Sum1/1
  Sum/1 -> prod3/3
  beta/1 -> Sum/1
  1-beta/1 -> Sum/2
  Sign/1 -> 1-beta/1
  prod4/1 -> Sign/1
  veloc/1 -> prod2/2, prod4/2
  prod1/1 -> force/1
  sliding friction/1 -> prod1/1

== system CSvRTHS_Client/simPC HC1/Offset/If Action ==
  In1 : Inport
  Action Port : ActionPort  PropagateVarSize=During execution  ActionPortLabel=if(u1 < nOffset)
  Data Store Read : DataStoreRead  DataStoreName=x0
  Data Store Write : DataStoreWrite  DataStoreName=x0
  Gain : Gain  Gain=1/nOffset  SaturateOnIntegerOverflow=on  OutDataTypeStr=Inherit: Same as input  ParamDataTypeStr=Inherit: Same as input
  Sum : Sum  Inputs=|++  InputSameDT=on  SaturateOnIntegerOverflow=on  OutDataTypeStr=Inherit: Same as first input
  wires:
  Data Store Read/1 -> Sum/2
  Sum/1 -> Data Store Write/1
  Gain/1 -> Sum/1
  In1/1 -> Gain/1

== system CSvRTHS_Client/simPC HC1/Offset1/If Action ==
  In1 : Inport
  Action Port : ActionPort  PropagateVarSize=During execution  ActionPortLabel=if(u1 < nOffset)
  Data Store Read : DataStoreRead  DataStoreName=x0
  Data Store Write : DataStoreWrite  DataStoreName=x0
  Gain : Gain  Gain=1/nOffset  SaturateOnIntegerOverflow=on  OutDataTypeStr=Inherit: Same as input  ParamDataTypeStr=Inherit: Same as input
  Sum : Sum  Inputs=|++  InputSameDT=on  SaturateOnIntegerOverflow=on  OutDataTypeStr=Inherit: Same as first input
  wires:
  Data Store Read/1 -> Sum/2
  Sum/1 -> Data Store Write/1
  Gain/1 -> Sum/1
  In1/1 -> Gain/1

== system CSvRTHS_Client/simPC HC1/SubSystem0/If Action Subsystem0 ==
  Action Port : ActionPort  PropagateVarSize=During execution  ActionPortLabel=if(u1 == 1)
  Data Store Write0 : DataStoreWrite  DataStoreName=sFlag
  Data Store Write1 : DataStoreWrite  DataStoreName=tFlag
  atTargetFlag : Constant  Value=0  OutDataTypeStr=int32  SampleTime=-1
  switchFlag : Constant  OutDataTypeStr=int32  SampleTime=-1
  wires:
  atTargetFlag/1 -> Data Store Write1/1
  switchFlag/1 -> Data Store Write0/1

== system CSvRTHS_Client/simPC HC1/SubSystem0/If Action Subsystem1 ==
  Action Port : ActionPort  PropagateVarSize=During execution  ActionPortLabel=if(u1 == 1)
  Data Store Write0 : DataStoreWrite  DataStoreName=sFlag
  switchFlag : Constant  Value=0  OutDataTypeStr=int32  SampleTime=-1
  wires:
  switchFlag/1 -> Data Store Write0/1

== system CSvRTHS_Client/simPC HC1/SubSystem1/For Each Subsystem ==
  i : Inport
  iDelay : Inport  Port=2  Partition=on  PartitionDimension=1  PartitionWidth=1  PartitionOffset=0
  measDsp : Inport  Port=3  Partition=on  PartitionDimension=1  PartitionWidth=1  PartitionOffset=0
  measFrc : Inport  Port=4  Partition=on  PartitionDimension=1  PartitionWidth=1  PartitionOffset=0
  For Each : ForEach  DisableCoverage=on
  SubSystem : Subsystem  TreatAsAtomicUnit=on
  Subsystem : Subsystem
  measDspOut : Outport  ConcatenationDimension=1
  measFrcOut : Outport  Port=2  ConcatenationDimension=1
  wires:
  Subsystem/1(trig) -> SubSystem/Trigger
  measDsp/1 -> SubSystem/1(measDsp In)
  measFrc/1 -> SubSystem/2(measFrc In)
  SubSystem/1(measDsp Out) -> measDspOut/1
  SubSystem/2(measFrc Out) -> measFrcOut/1
  iDelay/1 -> Subsystem/2(iDelay)
  i/1 -> Subsystem/1(i)

== system CSvRTHS_Client/simPC HC1/SubSystem1/SubSystem2 ==
  Trigger : TriggerPort  VariantControl=(inherit)
  Data Store Write : DataStoreWrite  DataStoreName=tFlag
  atTargetFlag : Constant  OutDataTypeStr=int32  SampleTime=-1
  wires:
  atTargetFlag/1 -> Data Store Write/1

== system CSvRTHS_Client/simPC HC1/SubSystem1/Subsystem2 ==
  i : Inport
  Add : Sum
  Constant : Constant  Value=max(iDelay)
  Constant1 : Constant  Value=N
  If : If  IfExpression=u1 == 0
  If Action Subsystem1 : Subsystem  TreatAsAtomicUnit=on
  If Action Subsystem2 : Subsystem  TreatAsAtomicUnit=on
  trig : Outport
  wires:
  Constant/1 -> If/1, If Action Subsystem2/2(In2)
  If/1 -> If Action Subsystem1/Action
  If/2 -> If Action Subsystem2/Action
  If Action Subsystem1/1(Out1) -> Add/1
  If Action Subsystem2/1(Out1) -> Add/2
  Add/1 -> trig/1
  i/1 -> If Action Subsystem1/2(In2), If Action Subsystem2/1(In1)
  Constant1/1 -> If Action Subsystem1/1(In1)

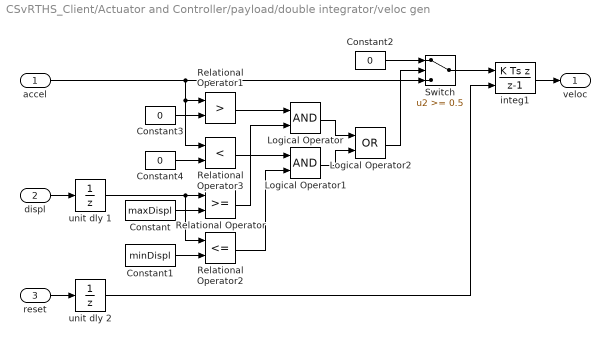
== system CSvRTHS_Client/Actuator and Controller/payload/double integrator/veloc gen ==
  accel : Inport
  displ : Inport  Port=2
  reset : Inport  Port=3
  Constant : Constant  Value=maxDispl
  Constant1 : Constant  Value=minDispl
  Constant2 : Constant  Value=0
  Constant3 : Constant  Value=0
  Constant4 : Constant  Value=0
  Logical Operator : Logic
  Logical Operator1 : Logic
  Logical Operator2 : Logic  Operator=OR
  Relational Operator : RelationalOperator  RndMeth=Nearest  InputSameDT=on
  Relational Operator1 : RelationalOperator  Operator=>  RndMeth=Nearest  InputSameDT=on
  Relational Operator2 : RelationalOperator  Operator=<=  RndMeth=Nearest  InputSameDT=on
  Relational Operator3 : RelationalOperator  Operator=<  RndMeth=Nearest  InputSameDT=on
  Switch : Switch  Threshold=0.5  SaturateOnIntegerOverflow=on  InputSameDT=on
  integ1 : DiscreteIntegrator  IntegratorMethod=Integration: Backward Euler  ExternalReset=either  SampleTime=0.5/1024  LimitOutput=on  UpperSaturationLimit=maxVeloc  LowerSaturationLimit=minVeloc  ICPrevOutput=DiscIntNeverNeededParam  ICPrevScaledInput=DiscIntNeverNeededParam
  unit dly 1 : UnitDelay  SampleTime=-1  HasFrameUpgradeWarning=on
  unit dly 2 : UnitDelay  SampleTime=-1  HasFrameUpgradeWarning=on
  veloc : Outport
  wires:
  integ1/1 -> veloc/1
  Constant/1 -> Relational Operator/2
  Relational Operator/1 -> Logical Operator/2
  Relational Operator2/1 -> Logical Operator1/2
  Constant1/1 -> Relational Operator2/2
  accel/1 -> Relational Operator3/1, Relational Operator1/1, Switch/3
  Constant3/1 -> Relational Operator1/2
  Relational Operator1/1 -> Logical Operator/1
  Constant4/1 -> Relational Operator3/2
  Relational Operator3/1 -> Logical Operator1/1
  Logical Operator/1 -> Logical Operator2/1
  Constant2/1 -> Switch/1
  Logical Operator2/1 -> Switch/2
  Switch/1 -> integ1/1
  unit dly 2/1 -> integ1/2
  Logical Operator1/1 -> Logical Operator2/2
  displ/1 -> unit dly 1/1
  reset/1 -> unit dly 2/1
  unit dly 1/1 -> Relational Operator/1, Relational Operator2/1

== system CSvRTHS_Client/simPC HC1/SubSystem1/For Each Subsystem/SubSystem ==
  measDsp In : Inport
  measFrc In : Inport  Port=2
  Trigger : TriggerPort  VariantControl=(inherit)
  measDsp Out : Outport  InitialOutput=[0]
  measFrc Out : Outport  Port=2  InitialOutput=[0]
  wires:
  measFrc In/1 -> measFrc Out/1
  measDsp In/1 -> measDsp Out/1

== system CSvRTHS_Client/simPC HC1/SubSystem1/For Each Subsystem/Subsystem ==
  i : Inport
  iDelay : Inport  Port=2
  Add : Sum
  Constant1 : Constant  Value=N
  If : If  IfExpression=u1 == 0
  If Action Subsystem1 : Subsystem  TreatAsAtomicUnit=on
  If Action Subsystem2 : Subsystem  TreatAsAtomicUnit=on
  trig : Outport
  wires:
  iDelay/1 -> If/1, If Action Subsystem2/2(In2)
  If/1 -> If Action Subsystem1/Action
  If/2 -> If Action Subsystem2/Action
  If Action Subsystem1/1(Out1) -> Add/1
  If Action Subsystem2/1(Out1) -> Add/2
  Add/1 -> trig/1
  i/1 -> If Action Subsystem1/2(In2), If Action Subsystem2/1(In1)
  Constant1/1 -> If Action Subsystem1/1(In1)

== system CSvRTHS_Client/simPC HC1/SubSystem1/Subsystem2/If Action Subsystem1 ==
  In1 : Inport
  In2 : Inport  Port=2
  Action Port : ActionPort  ActionPortLabel=if(u1 == 0)
  Relational Operator : RelationalOperator  Operator===  OutDataTypeStr=boolean  RndMeth=Nearest
  Out1 : Outport
  wires:
  Relational Operator/1 -> Out1/1
  In1/1 -> Relational Operator/1
  In2/1 -> Relational Operator/2

== system CSvRTHS_Client/simPC HC1/SubSystem1/Subsystem2/If Action Subsystem2 ==
  In1 : Inport
  In2 : Inport  Port=2
  Action Port : ActionPort  ActionPortLabel=else
  Relational Operator : RelationalOperator  Operator===  OutDataTypeStr=boolean  RndMeth=Nearest
  Out1 : Outport
  wires:
  Relational Operator/1 -> Out1/1
  In1/1 -> Relational Operator/1
  In2/1 -> Relational Operator/2

== system CSvRTHS_Client/simPC HC1/SubSystem1/For Each Subsystem/Subsystem/If Action Subsystem1 ==
  In1 : Inport
  In2 : Inport  Port=2
  Action Port : ActionPort  ActionPortLabel=if(u1 == 0)
  Relational Operator : RelationalOperator  Operator===  OutDataTypeStr=boolean  RndMeth=Nearest
  Out1 : Outport
  wires:
  Relational Operator/1 -> Out1/1
  In1/1 -> Relational Operator/1
  In2/1 -> Relational Operator/2

== system CSvRTHS_Client/simPC HC1/SubSystem1/For Each Subsystem/Subsystem/If Action Subsystem2 ==
  In1 : Inport
  In2 : Inport  Port=2
  Action Port : ActionPort  ActionPortLabel=else
  Relational Operator : RelationalOperator  Operator===  OutDataTypeStr=boolean  RndMeth=Nearest
  Out1 : Outport
  wires:
  Relational Operator/1 -> Out1/1
  In1/1 -> Relational Operator/1
  In2/1 -> Relational Operator/2

== stateflow chart CSvRTHS_Client/simPC HC1/Predictor-Corrector ==
  state HybridController [parallel]
    settings: executionOrder=1
    state Correct
      en: state = 0;
      en: setCurSig(comD,i/N);
      en: targLocal = targD; setNewSig(targLocal);
      en: di = min(max(diSD+1/(0.2*N)*(i-iSD),0.001),1.0);
      en: i = min(i+di,N);
      en: correctD2(comD,i/N);
      en: correctV2(comV,i/N); correctA2(comA,i/N);
      du: di = min(max(diSD+1/(0.2*N)*(i-iSD),0.001),1.0);
      du: i = min(i+di,N);
      du: correctD2(comD,i/N);
      du: correctV2(comV,i/N); correctA2(comA,i/N);
    state Predict
      en: state = 1;
      en: setCurSig(comD,1.0);
      en: i = 1; iSD = 0; diSD = 1;
      en: predictD2(comD,i/N);
      en: predictV2(comV,i/N); predictA2(comA,i/N);
      du: i++;
      du: predictD2(comD,i/N);
      du: predictV2(comV,i/N); predictA2(comA,i/N);
    state Initialize
      en: i = 0; iSD = 0; diSD = 1;
      en: initData(nDOF,dtCon,dtSim,dtInt);
      en: zeroSig(comD);
      en: zeroSig(comV);
      en: zeroSig(comA);
    state AutoSlowDown
      en: state = 2;
      en: diSD = 4-i/(0.2*N);
      en: i += diSD; iSD = i;
      en: predictD2(comD,i/N);
      en: predictV2(comV,i/N); predictA2(comA,i/N);
      du: diSD = 4-i/(0.2*N);
      du: i += diSD; iSD = i;
      du: predictD2(comD,i/N);
      du: predictV2(comV,i/N); predictA2(comA,i/N);
    Correct -> Predict [order 1] : [i>=N && flag!=1]
    (default) -> Initialize
    Initialize -> Correct : [flag==1]
    Predict -> Correct [order 2] : [flag==1]
    Predict -> AutoSlowDown [order 1] : [i>=0.6*N && flag!=1]
    AutoSlowDown -> Correct : [flag==1]
    Correct -> Correct [order 2] : [flag==1]
        | {i=0; iSD=0; diSD=1}
  data: targD input double size=nDOF+1; flag input int32; comD output double size=nDOF+1; comV output double size=nDOF+1; comA output double size=nDOF+1; state output int32; i output double; N parameter int32; nDOF parameter int32; di local double; diSD local double; iSD local double; targLocal local double size=nDOF+1; dtCon parameter double; dtSim parameter double; dtInt parameter double

== matlab function CSvRTHS_Client/MCB/Gradient Adaptive Law/gradiente_adaptive_law ==
  data: x_m input; x_c input; amb_a input; A_ambp output; adaptivegain input
function A_ambp   = fcn(x_m,x_c,amb_a,adaptivegain)
error=(x_c-amb_a'*x_m)/(1+(x_m'*x_m));
A_ambp=adaptivegain*error*x_m;
